simulink library "lowFreqWithFAUTurb_cl"  (R2018b)
settings: Solver=VariableStepAuto  StartTime=0.0  StopTime=10.0  RelTol=1e-3
libraries: highFreqFlowData_ul x1, lowFreqFlowData_ul x1
settings Model: Creator=jcreed2  LastModifiedBy=mcobb

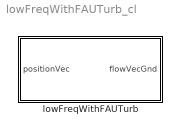
== system lowFreqWithFAUTurb_cl ==
  lowFreqWithFAUTurb : Subsystem

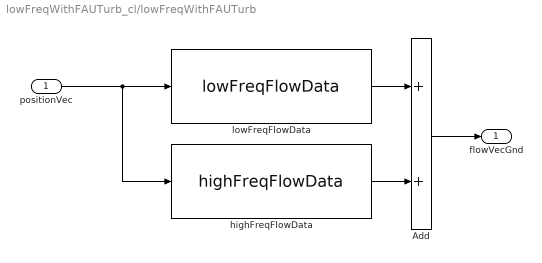
== system lowFreqWithFAUTurb_cl/lowFreqWithFAUTurb ==
  positionVec : Inport
  Add : Sum
  highFreqFlowData : highFreqFlowData_ul/highFreqFlowData  SystemSampleTime=-1
  lowFreqFlowData : lowFreqFlowData_ul/lowFreqFlowData  SystemSampleTime=-1  VariantControl=VSS_flowCalculation_constXYZT
  flowVecGnd : Outport
  wires:
  positionVec/1 -> highFreqFlowData/1, lowFreqFlowData/1
  lowFreqFlowData/1 -> Add/1
  highFreqFlowData/1 -> Add/2
  Add/1 -> flowVecGnd/1
